simulink model "three_phase_circuit_Sim01"  (R2020b)
settings: Solver=ode4  StartTime=0.0  StopTime=inf  FixedStep=Ts  RelTol=1e-3  EnableMultiTasking=on
PostLoadFcn:
  | Ts=75e-6;
InitFcn:
  | Ts=75e-6;
undefined symbols (not defined in the file): IP, j, UDP
libraries: powerlib x40, simulink x6, powerlib_meascontrol x6, rtlab x5, rtio_generic_ip x1
Description:
  | Model of a simple control system for use iin training.
settings Model: Creator=Paul Baracos  LastModifiedBy=Antero
settings DataIOCC: LimitDataPoints=on  SaveFormat=Array  SignalLoggingSaveFormat=ModelDataLogs  SaveOutput=off  SaveTime=off  ReturnWorkspaceOutputs=off  SignalLoggingName=sigsOut
settings OptimizationCC: BlockReduction=off  BooleanDataType=off  OptimizeBlockIOStorage=off  BufferReuse=off  ExpressionFolding=off  LocalBlockOutputs=off  InitFltsAndDblsToZero=on  LifeSpan=inf
settings DebuggingCC: SaveWithParameterizedLinksMsg=none  UnderspecifiedInitializationDetection=Classic  MergeDetectMultiDrivingBlocksExec=none  SignalResolutionControl=TryResolveAllWithWarning  MultiTaskDSMMsg=warning  MultiTaskCondExecSysMsg=none  FcnCallInpInsideContextMsg=warning  SFUnexpectedBacktrackingDiag=warning  SFNoUnconditionalDefaultTransitionDiag=warning  SFExecutionAtInitializationDiag=none  ArithmeticOperatorsInVariantConditions=warning
settings HardwareCC: ProdBitPerPointer=32  ProdBitPerSizeT=32  ProdBitPerPtrDiffT=32  ProdLargestAtomicFloat=None  ProdIntDivRoundTo=Undefined  ProdEndianess=Unspecified  ProdWordSize=32  ProdHWDeviceType=32-bit Generic  TargetBitPerPointer=64  TargetBitPerSizeT=64  TargetBitPerPtrDiffT=64  TargetLongLongMode=on  TargetIntDivRoundTo=Zero  TargetEndianess=LittleEndian  TargetWordSize=64  TargetHWDeviceType=MATLAB Host  ProdEqTarget=off
settings ModelReferenceCC: PropagateSignalLabelsOutOfModel=off
settings SFSimCC: SimUseLocalCustomCode=off  CustomCodeUndefinedFunction=UseInterfaceOnly
settings RTWCC: RTWUseLocalCustomCode=off
settings CodeAppCC: StateflowObjectComments=on
settings GRTTargetCC: TargetFcnLib=ansi_tfl_tmw.mat  TargetLangStandard=C89/C90 (ANSI)  CombineOutputUpdateFcns=off  GRTInterface=on
settings ConfigComp: CovMetricSettings=dw  CovSaveCumulativeToWorkspaceVar=on  CovSaveSingleToWorkspaceVar=on  CovExternalEMLEnable=off

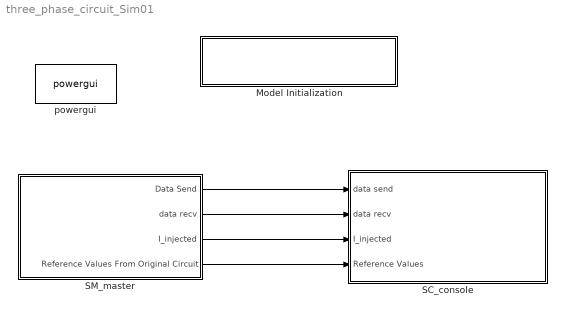
== system three_phase_circuit_Sim01 ==
  Model Initialization : Subsystem  AncestorBlock=artemis/Tools /Misc/Model Initialization  mask(Model Functions){InitFcnX=Ts=75e-6;, prel=off, posl=on, inif=on, strf=off}
      mask prompts: InitFcnX "Initialisation"; prel "Preload Function"; posl "PostLoad Function"; inif "InitFcn"; strf "StartFcn"
      mask init:
      | currentBlock = gcb;
      | root = bdroot(currentBlock);
      | 
      | if ~strcmp(get_param(root,'BlockDiagramType'),'library')
      |     if prel==1
      |         set_param(root, 'PreLoadFcn', InitFcnX);
      |     else
      |         set_param(root, 'PreLoadFcn', '');
      |     end
      |     if inif==1
      |         set_param(root, 'InitFcn', InitFcnX);
      |     else
      |         set_param(root, 'InitFcn', '');
      |     end
      |     if strf==1
      |         set_param(root, 'StartFcn', InitFcnX);
      |     else
      |         set_param(root, 'StartFcn', '');
      |     end
      |     if posl==1
      |         set_param(root, 'PostLoadFcn', InitFcnX);
      |     else
      |         set_param(root, 'PostLoadFcn', '');
      |     end
      | end
      | 
      | pos = get_param(currentBlock, 'Position');
      | width = pos(3) - pos(1); height = pos(4) - pos(2);
      | txt = [ upper(root) '\n' '- InitFcn. . . . . '  get_param(root, 'InitFcn') ];
      settings: CopyFcn=set_param(gcb,'LinkStatus','inactive')
      mask Display: text(5, height*0.5, txt, 'horizontalAlignment', 'left', 'verticalAlignment', 'middle') ;
  SC_console : Subsystem
  SM_master : Subsystem
  powergui : powerlib/powergui  Priority=1  SimulationMode=Discrete  SampleTime=Ts  frequency=60  Iterations=50  frequencyindice=60  Pbase=100e6  ErrMax=1e-4  UnitsV=kV  UnitsW=MW  buscounter=0  FunctionMessages=off  echomessages=off  EnableUseOfTLC=off  CurrentSourceSwitches=off  DisableSnubberDevices=off  DisableRonSwitches=off  DisableVfSwitches=off  DisplayEquations=off  AutomaticDiscreteSolvers=off  SolverType=Tustin/Backward Euler (TBE)  Interpol=off  ExternalGateDelay=off  methode=off  Ts=100  x0status=blocks  SPID=on  SwTol=0  HookPort=off  NonlinearTolerance=1e-4  nMaxIteration=100  ContinueOnMaxIteration=off  RestoreLinks=warning  ResistiveCurrentMeasurement=off  Frange=[0:2:500]  Ylog=off  Xlog=on  ShowGrid=off  save=off  variable=ZData  structure=0  ZoomFFT=off  StartTime=0.0  cycles=1  DisplayStyle=1  fundamental=60  FreqAxis=off  MaxFrequency=1000  frequencyindicesteady=1  RmsSteady=1  display=off
  wires:
  SM_master/1(Data Send) -> SC_console/1(data send)
  SM_master/3(I_injected) -> SC_console/3(I_injected)
  SM_master/2(data recv) -> SC_console/2(data recv)
  SM_master/4(Reference Values From Original Circuit) -> SC_console/4(Reference Values)

== system three_phase_circuit_Sim01/Model Initialization ==

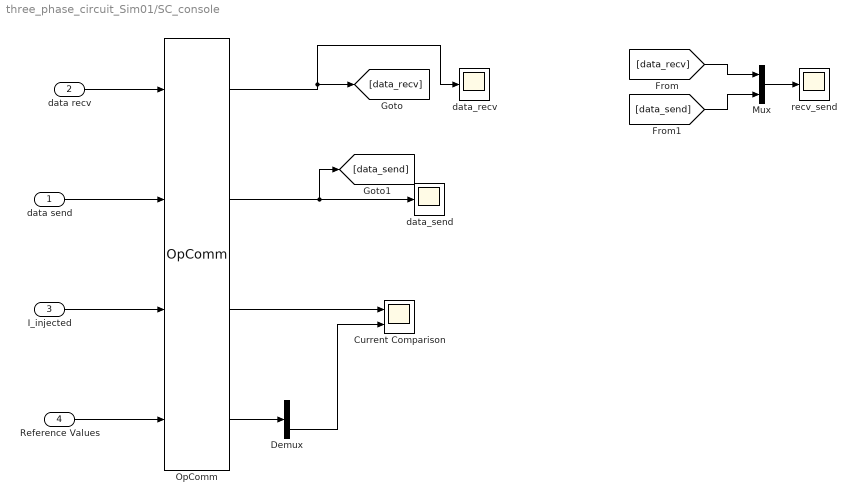
== system three_phase_circuit_Sim01/SC_console ==
  data send : Inport
  data recv : Inport  Port=2
  I_injected : Inport  Port=3
  Reference Values : Inport  Port=4
  Current Comparison : Scope  NumInputPorts=2
  Demux : Demux  Outputs=2
  Mux : Mux  Inputs=2
  OpComm : rtlab/OpComm  nbport=4  groupe_acq=1  subsys_rate=0  st=0  Synchronization=on  Interpolation=on  Threshold=1.0  Missed_Data=off  Sim_Time=off  Samples=off  dynSigOut=off  from_console=0  warning_done=off  writeOpCommFile=off  Offset=off
      settings: SourceProductName=RT-LAB
  data_recv : Scope
  data_send : Scope
  recv_send : Scope
  wires:
  OpComm/2 -> [data_send], data_send/1
  data recv/1 -> OpComm/1
  [data_recv] -> Mux/1
  OpComm/1 -> data_recv/1, [data_recv]
  Reference Values/1 -> OpComm/4
  Mux/1 -> recv_send/1
  OpComm/3 -> Current Comparison/1
  data send/1 -> OpComm/2
  I_injected/1 -> OpComm/3
  [data_send] -> Mux/2
  OpComm/4 -> Demux/1
  Demux/2 -> Current Comparison/2

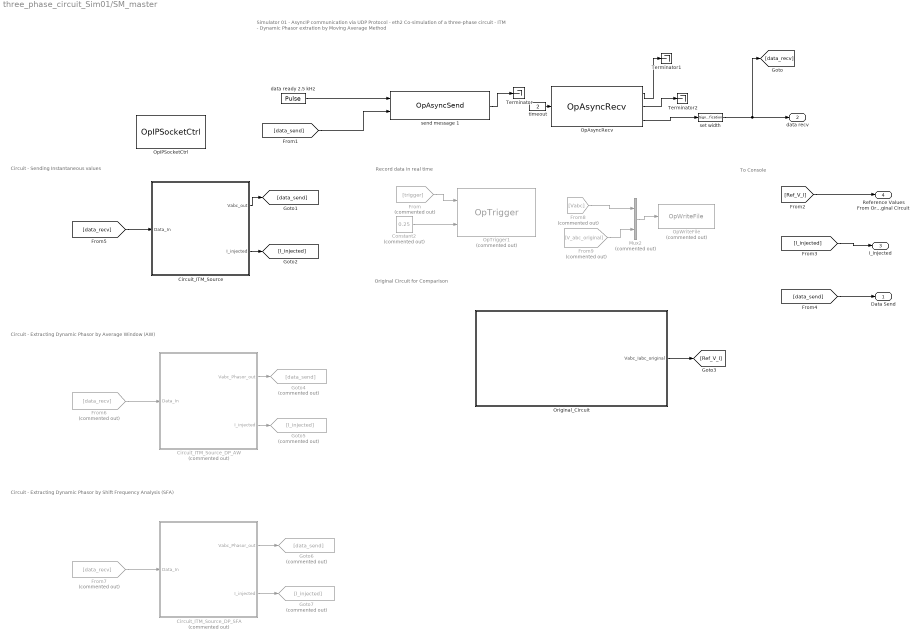
== system three_phase_circuit_Sim01/SM_master ==
  note: To Console
  note: Original Circuit for Comparison
  note: Simulator 01 - AsyncIP communication via UDP Protocol - eth2
      |
      | Co-simulation of a three-phase circuit - ITM - Dynamic Phasor extration by Moving Average Method
  note: Circuit - Sending Instantaneous values
  note: Circuit - Extracting Dynamic Phasor by Average Window (AW)
  note: Circuit - Extracting Dynamic Phasor by Shift Frequency Analysis (SFA)
  note: Record data in real time
  Circuit_ITM_Source : Subsystem
  Circuit_ITM_Source_DP_AW : Subsystem  Commented=on
  Circuit_ITM_Source_DP_SFA : Subsystem  Commented=on
  Constant2 : Constant  Commented=on  Value=0.25
  From : From  Commented=on  GotoTag=trigger
  From6 : From  Commented=on  GotoTag=data_recv
  From7 : From  Commented=on  GotoTag=data_recv
  From8 : From  Commented=on  GotoTag=Vabc
  From9 : From  Commented=on  GotoTag=V_abc_original
  Goto4 : Goto  Commented=on  GotoTag=data_send
  Goto5 : Goto  Commented=on  GotoTag=I_injected
  Goto6 : Goto  Commented=on  GotoTag=data_send
  Goto7 : Goto  Commented=on  GotoTag=I_injected
  Mux2 : Mux  Commented=on  Inputs=2
  OpAsyncRecv : rtlab/Communication/Asynchronous/OpAsyncRecv  ctl_id=1  recv_id=1  enable_param=off  fp1=1  fp2=2  fp3=3  fp4=4  fp5=5  sp1=string1  sp2=string2  sp3=string3  sp4=string4  sp5=string5  fp6=6  fp7=7
      settings: SourceProductName=RT-LAB
  OpIPSocketCtrl : rtio_generic_ip/OpIPSocketCtrl  ctl_id=1  proto=UDP/IP  ip_addr_remote=192.168.0.232  ip_port_remote=25000  ip_port_local=0  ip_addr_mcast=0.0.0.0  exe_name=AsyncIP
      settings: SourceProductName=RT-LAB I/O
  OpTrigger1 : rtlab/DataLogging/OpTrigger  Commented=on  Trig_Type=RISING EDGE  Trig_Offset=0  Acq_Group=26
      settings: SourceProductName=RT-LAB
  OpWriteFile : rtlab/DataLogging/OpWriteFile  Commented=on  Static_File=on  varname=data_voltage  Filename=data_sim02.mat  rtpath='./'  nrtpath='.\'  Acq_Group=26  file_size=8640000  write_offline=off  Sim_Mode=off  Nb_Samples=100000  Buffer_size=2400000
      settings: SourceProductName=RT-LAB
  Original_Circuit : Subsystem
  Terminator : Terminator
  Terminator1 : Terminator
  Terminator2 : Terminator
  data ready 2.5 kHz : DiscretePulseGenerator  PulseWidth=2  SampleTime=Ts
  send message 1 : rtlab/Communication/Asynchronous/OpAsyncSend  ctl_id=1  send_id=1  mode=DONT_NEED_REPLY  enable_param=off  fp1=1  fp2=2  fp3=3  fp4=4  fp5=5  sp1=string1  sp2=string2  sp3=string3  sp4=string4  sp5=string5
      settings: SourceProductName=RT-LAB
  set width : SignalSpecification  Dimensions=3  SampleTime=Ts
  timeout : Constant  Value=2
  Data Send : Outport
  data recv : Outport  Port=2
  I_injected : Outport  Port=3
  Reference Values From Original Circuit : Outport  Port=4
  wires:
  OpAsyncRecv/3 -> set width/1
  timeout/1 -> OpAsyncRecv/1
  data ready 2.5 kHz/1 -> send message 1/1
  OpAsyncRecv/1 -> Terminator1/1
  OpAsyncRecv/2 -> Terminator2/1
  set width/1 -> [data_recv], data recv/1
  [data_send] -> send message 1/2
  send message 1/1 -> Terminator/1
  [data_recv] -> Circuit_ITM_Source/1(Data_In)
  Circuit_ITM_Source/1(Vabc_out) -> [data_send]
  Circuit_ITM_Source/2(I_injected) -> [I_injected]
  [Ref_V_I] -> Reference Values From Original Circuit/1
  [I_injected] -> I_injected/1
  [data_send] -> Data Send/1
  Circuit_ITM_Source_DP_AW/2(I_injected) -> Goto5/1
  Circuit_ITM_Source_DP_AW/1(Vabc_Phasor_out) -> Goto4/1
  From6/1 -> Circuit_ITM_Source_DP_AW/1(Data_In)
  From7/1 -> Circuit_ITM_Source_DP_SFA/1(Data_In)
  Circuit_ITM_Source_DP_SFA/1(Vabc_Phasor_out) -> Goto6/1
  Original_Circuit/1(Vabc_Iabc_original) -> [Ref_V_I]
  Circuit_ITM_Source_DP_SFA/2(I_injected) -> Goto7/1
  Mux2/1 -> OpWriteFile/1
  From/1 -> OpTrigger1/1
  Constant2/1 -> OpTrigger1/2
  From9/1 -> Mux2/2
  From8/1 -> Mux2/1

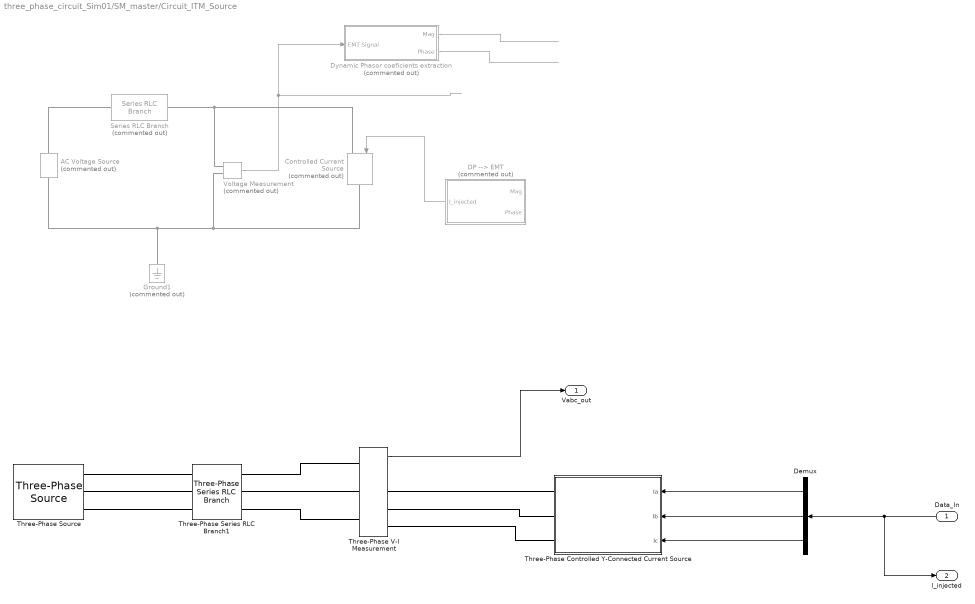
== system three_phase_circuit_Sim01/SM_master/Circuit_ITM_Source ==
  Data_In : Inport
  AC Voltage Source : powerlib/Electrical Sources/AC Voltage Source  Commented=on  Amplitude=100  Phase=0  Frequency=60  SampleTime=0  Measurements=None  BusType=swing  Pref=10e3  Qref=0  Qmin=-inf  Qmax=+inf
  Controlled Current Source : powerlib/Electrical Sources/Controlled Current Source  Commented=on  Initialize=on  Source_Type=AC  Amplitude=0  Phase=0  Frequency=0  Measurements=None
  DP --> EMT : Subsystem  Commented=on
  Demux : Demux  Outputs=3
  Dynamic Phasor coeficients extraction : Subsystem  Commented=on
  Ground1 : powerlib/Elements/Ground  Commented=on  LConnTagsString=a
  Series RLC Branch : powerlib/Elements/Series RLC Branch  Commented=on  LConnTagsString=__new0  RConnTagsString=__new0  BranchType=R  Resistance=0.5  Inductance=1e-3  SetiL0=off  InitialCurrent=0  Capacitance=1e-6  Setx0=off  InitialVoltage=0  Measurements=None
  Three-Phase Series RLC Branch1 : powerlib/Elements/Three-Phase Series RLC Branch  LConnTagsString=A|B|C  RConnTagsString=A|B|C  BranchType=R  Resistance=2  Inductance=1e-3  Capacitance=1e-6  Measurements=None
  Three-Phase V-I Measurement : powerlib/Measurements/Three-Phase V-I Measurement  VoltageMeasurement=phase-to-ground  SetLabelV=off  LabelV=Vabc  Vpu=off  VpuLL=off  CurrentMeasurement=yes  SetLabelI=off  LabelI=Iabc  Ipu=off  Pbase=100e6  Vbase=25e3  OutputType=Complex  PhasorSimulation=off  PSBequivalent=0
  Three-Phase Controlled Y-Connected Current Source : Subsystem
      settings: PortSchema="{\"entries\":[{\"content\":{\"sides\":[{\"content\":{\"connectorIds\":[\"LConn1\",\"LConn2\",\"LConn3\"]},\"type\":\"ConnectorPlacement.EquallySpacedRectSide\",\"uuid\":\"a8a67328-a09d-4495-b33c-aaf3ca0795cb\"},{\"content\":{\"connectorIds\":[\"In1\",\"In2\",\"In3\"],\"side\":\"RIGHT\"},\"type\":\"ConnectorPlacement.EquallySpacedRectSide\",\"uuid\":\"ca8d97e2-0dea-49aa-8cb7-235b4eace1f8\"},{\"content\":{\"connectorIds\":[],\"side\":\"TOP\"},\"type\":\"ConnectorPlacement.EquallySpacedRectSide\",\"uuid\":\"ab6aade9-1d27-4135-8ce1-c4358d4ecc87\"}]},\"type\":\"ConnectorPlacement.EquallySpacedConnector\",\"uuid\":\"205b5c38-55ea-4d68-a706-de660c21807c\"}],\"packageUris\":[\"http://schema.mathworks.com/mf0/Connector/19700101\"],\"version\":\"1.0\"}"
  Three-Phase Source : powerlib/Electrical Sources/Three-Phase Source  InternalConnection=Yg  VoltagePhases=off  Voltage=220  PhaseAngle=0  Voltage_phases=[25e3 25e3 25e3]/sqrt(3)  PhaseAngles_phases=[0 -120 +120]  Frequency=60  NonIdealSource=on  SpecifyImpedance=off  Resistance=0  Inductance=0  ShortCircuitLevel=100e6  BaseVoltage=220  XRratio=7  BusType=swing  Pref=10e3  Qref=0  Prefabc=[10e3, 10e3, 10e3]  Qrefabc=[0, 0, 0]  Qmin=-inf  Qmax=inf
  Voltage Measurement : powerlib/Measurements/Voltage Measurement  Commented=on  PhasorSimulation=off  OutputType=Complex  PSBequivalent=0
  Vabc_out : Outport
  I_injected : Outport  Port=2
  wires:
  DP --> EMT/1(I_injected) -> Controlled Current Source/1
  Voltage Measurement/1 -> Dynamic Phasor coeficients extraction/1(EMT Signal)
  Dynamic Phasor coeficients extraction/1(Mag) -> ?
  Dynamic Phasor coeficients extraction/2(Phase) -> ?
  Demux/1 -> Three-Phase Controlled Y-Connected Current Source/1(Ia)
  Demux/2 -> Three-Phase Controlled Y-Connected Current Source/2(Ib)
  Demux/3 -> Three-Phase Controlled Y-Connected Current Source/3(Ic)
  Data_In/1 -> Demux/1, I_injected/1
  Three-Phase V-I Measurement/1 -> Vabc_out/1
  connections:
  AC Voltage Source/RConn1 -- Series RLC Branch/LConn1
  AC Voltage Source/LConn1 -- Controlled Current Source/RConn1 -- Voltage Measurement/LConn2 -- Ground1/LConn1
  Series RLC Branch/RConn1 -- Voltage Measurement/LConn1 -- Controlled Current Source/LConn1
  Three-Phase Series RLC Branch1/LConn3 -- Three-Phase Source/RConn3
  Three-Phase Series RLC Branch1/RConn2 -- Three-Phase V-I Measurement/LConn2
  Three-Phase V-I Measurement/LConn3 -- Three-Phase Series RLC Branch1/RConn3
  Three-Phase Source/RConn1 -- Three-Phase Series RLC Branch1/LConn1
  Three-Phase V-I Measurement/LConn1 -- Three-Phase Series RLC Branch1/RConn1
  Three-Phase Source/RConn2 -- Three-Phase Series RLC Branch1/LConn2
  Three-Phase Controlled Y-Connected Current Source/LConn1 -- Three-Phase V-I Measurement/RConn1
  Three-Phase V-I Measurement/RConn2 -- Three-Phase Controlled Y-Connected Current Source/LConn2
  Three-Phase V-I Measurement/RConn3 -- Three-Phase Controlled Y-Connected Current Source/LConn3

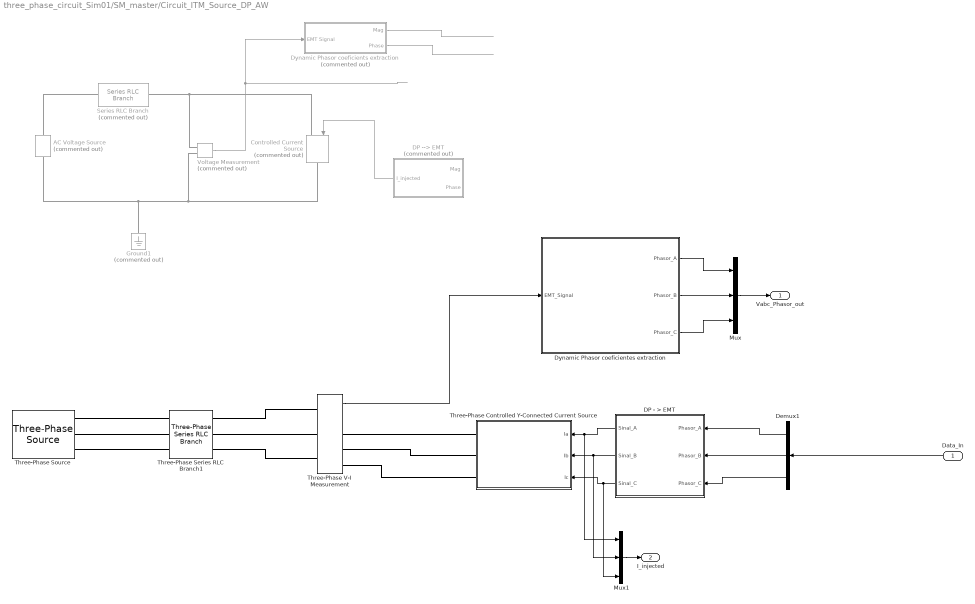
== system three_phase_circuit_Sim01/SM_master/Circuit_ITM_Source_DP_AW ==
  Data_In : Inport
  AC Voltage Source : powerlib/Electrical Sources/AC Voltage Source  Commented=on  Amplitude=100  Phase=0  Frequency=60  SampleTime=0  Measurements=None  BusType=swing  Pref=10e3  Qref=0  Qmin=-inf  Qmax=+inf
  Controlled Current Source : powerlib/Electrical Sources/Controlled Current Source  Commented=on  Initialize=on  Source_Type=AC  Amplitude=0  Phase=0  Frequency=0  Measurements=None
  DP - > EMT : Subsystem
  DP --> EMT : Subsystem  Commented=on
  Demux1 : Demux  Outputs=3
  Dynamic Phasor coeficientes extraction : Subsystem
  Dynamic Phasor coeficients extraction : Subsystem  Commented=on
  Ground1 : powerlib/Elements/Ground  Commented=on  LConnTagsString=a
  Mux : Mux  Inputs=3
  Mux1 : Mux  Inputs=3
  Series RLC Branch : powerlib/Elements/Series RLC Branch  Commented=on  LConnTagsString=__new0  RConnTagsString=__new0  BranchType=R  Resistance=0.5  Inductance=1e-3  SetiL0=off  InitialCurrent=0  Capacitance=1e-6  Setx0=off  InitialVoltage=0  Measurements=None
  Three-Phase Series RLC Branch1 : powerlib/Elements/Three-Phase Series RLC Branch  LConnTagsString=A|B|C  RConnTagsString=A|B|C  BranchType=R  Resistance=2  Inductance=1e-3  Capacitance=1e-6  Measurements=None
  Three-Phase V-I Measurement : powerlib/Measurements/Three-Phase V-I Measurement  VoltageMeasurement=phase-to-ground  SetLabelV=off  LabelV=Vabc  Vpu=off  VpuLL=off  CurrentMeasurement=yes  SetLabelI=off  LabelI=Iabc  Ipu=off  Pbase=100e6  Vbase=25e3  OutputType=Complex  PhasorSimulation=off  PSBequivalent=0
  Three-Phase Controlled Y-Connected Current Source : Subsystem
      settings: PortSchema="{\"entries\":[{\"content\":{\"sides\":[{\"content\":{\"connectorIds\":[\"LConn1\",\"LConn2\",\"LConn3\"]},\"type\":\"ConnectorPlacement.EquallySpacedRectSide\",\"uuid\":\"a8a67328-a09d-4495-b33c-aaf3ca0795cb\"},{\"content\":{\"connectorIds\":[\"In1\",\"In2\",\"In3\"],\"side\":\"RIGHT\"},\"type\":\"ConnectorPlacement.EquallySpacedRectSide\",\"uuid\":\"ca8d97e2-0dea-49aa-8cb7-235b4eace1f8\"},{\"content\":{\"connectorIds\":[],\"side\":\"TOP\"},\"type\":\"ConnectorPlacement.EquallySpacedRectSide\",\"uuid\":\"ab6aade9-1d27-4135-8ce1-c4358d4ecc87\"}]},\"type\":\"ConnectorPlacement.EquallySpacedConnector\",\"uuid\":\"205b5c38-55ea-4d68-a706-de660c21807c\"}],\"packageUris\":[\"http://schema.mathworks.com/mf0/Connector/19700101\"],\"version\":\"1.0\"}"
  Three-Phase Source : powerlib/Electrical Sources/Three-Phase Source  InternalConnection=Yg  VoltagePhases=off  Voltage=220  PhaseAngle=0  Voltage_phases=[25e3 25e3 25e3]/sqrt(3)  PhaseAngles_phases=[0 -120 +120]  Frequency=60  NonIdealSource=on  SpecifyImpedance=off  Resistance=0  Inductance=0  ShortCircuitLevel=100e6  BaseVoltage=220  XRratio=7  BusType=swing  Pref=10e3  Qref=0  Prefabc=[10e3, 10e3, 10e3]  Qrefabc=[0, 0, 0]  Qmin=-inf  Qmax=inf
  Voltage Measurement : powerlib/Measurements/Voltage Measurement  Commented=on  PhasorSimulation=off  OutputType=Complex  PSBequivalent=0
  Vabc_Phasor_out : Outport
  I_injected : Outport  Port=2
  wires:
  DP --> EMT/1(I_injected) -> Controlled Current Source/1
  Voltage Measurement/1 -> Dynamic Phasor coeficients extraction/1(EMT Signal)
  Dynamic Phasor coeficients extraction/1(Mag) -> ?
  Dynamic Phasor coeficients extraction/2(Phase) -> ?
  Data_In/1 -> Demux1/1
  Three-Phase V-I Measurement/1 -> Dynamic Phasor coeficientes extraction/1(EMT_Signal)
  Dynamic Phasor coeficientes extraction/3(Phasor_C) -> Mux/3
  Dynamic Phasor coeficientes extraction/2(Phasor_B) -> Mux/2
  Dynamic Phasor coeficientes extraction/1(Phasor_A) -> Mux/1
  Mux/1 -> Vabc_Phasor_out/1
  Demux1/1 -> DP - > EMT/1(Phasor_A)
  Demux1/2 -> DP - > EMT/2(Phasor_B)
  Demux1/3 -> DP - > EMT/3(Phasor_C)
  DP - > EMT/2(Sinal_B) -> Mux1/2, Three-Phase Controlled Y-Connected Current Source/2(Ib)
  DP - > EMT/1(Sinal_A) -> Mux1/1, Three-Phase Controlled Y-Connected Current Source/1(Ia)
  DP - > EMT/3(Sinal_C) -> Mux1/3, Three-Phase Controlled Y-Connected Current Source/3(Ic)
  Mux1/1 -> I_injected/1
  connections:
  AC Voltage Source/RConn1 -- Series RLC Branch/LConn1
  AC Voltage Source/LConn1 -- Controlled Current Source/RConn1 -- Voltage Measurement/LConn2 -- Ground1/LConn1
  Series RLC Branch/RConn1 -- Voltage Measurement/LConn1 -- Controlled Current Source/LConn1
  Three-Phase Series RLC Branch1/LConn3 -- Three-Phase Source/RConn3
  Three-Phase Series RLC Branch1/RConn2 -- Three-Phase V-I Measurement/LConn2
  Three-Phase V-I Measurement/LConn3 -- Three-Phase Series RLC Branch1/RConn3
  Three-Phase Source/RConn1 -- Three-Phase Series RLC Branch1/LConn1
  Three-Phase V-I Measurement/LConn1 -- Three-Phase Series RLC Branch1/RConn1
  Three-Phase Source/RConn2 -- Three-Phase Series RLC Branch1/LConn2
  Three-Phase Controlled Y-Connected Current Source/LConn1 -- Three-Phase V-I Measurement/RConn1
  Three-Phase V-I Measurement/RConn2 -- Three-Phase Controlled Y-Connected Current Source/LConn2
  Three-Phase V-I Measurement/RConn3 -- Three-Phase Controlled Y-Connected Current Source/LConn3

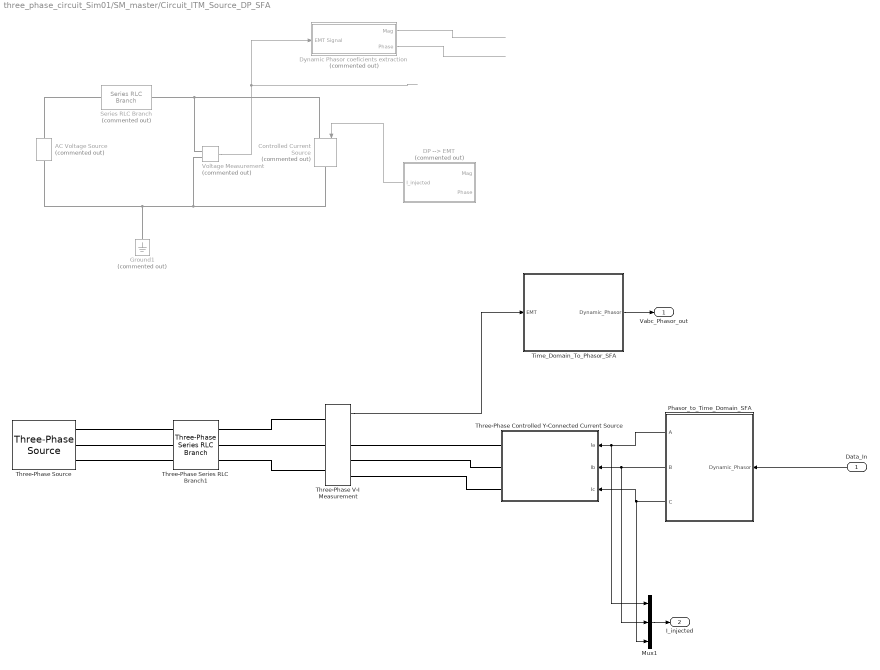
== system three_phase_circuit_Sim01/SM_master/Circuit_ITM_Source_DP_SFA ==
  Data_In : Inport
  AC Voltage Source : powerlib/Electrical Sources/AC Voltage Source  Commented=on  Amplitude=100  Phase=0  Frequency=60  SampleTime=0  Measurements=None  BusType=swing  Pref=10e3  Qref=0  Qmin=-inf  Qmax=+inf
  Controlled Current Source : powerlib/Electrical Sources/Controlled Current Source  Commented=on  Initialize=on  Source_Type=AC  Amplitude=0  Phase=0  Frequency=0  Measurements=None
  DP --> EMT : Subsystem  Commented=on
  Dynamic Phasor coeficients extraction : Subsystem  Commented=on
  Ground1 : powerlib/Elements/Ground  Commented=on  LConnTagsString=a
  Mux1 : Mux  Inputs=3
  Phasor_to_Time_Domain_SFA : Subsystem  mask(Time domain from Dynamic Phasor){offset=60}
      mask prompts: offset "Frequency shift"
      mask help: This block extracts Time Domain Signals from the Dynamic Phasor by using the SFA method. It is usable only for three-phase signals
  Series RLC Branch : powerlib/Elements/Series RLC Branch  Commented=on  LConnTagsString=__new0  RConnTagsString=__new0  BranchType=R  Resistance=0.5  Inductance=1e-3  SetiL0=off  InitialCurrent=0  Capacitance=1e-6  Setx0=off  InitialVoltage=0  Measurements=None
  Three-Phase Series RLC Branch1 : powerlib/Elements/Three-Phase Series RLC Branch  LConnTagsString=A|B|C  RConnTagsString=A|B|C  BranchType=R  Resistance=2  Inductance=1e-3  Capacitance=1e-6  Measurements=None
  Three-Phase V-I Measurement : powerlib/Measurements/Three-Phase V-I Measurement  VoltageMeasurement=phase-to-ground  SetLabelV=off  LabelV=Vabc  Vpu=off  VpuLL=off  CurrentMeasurement=yes  SetLabelI=off  LabelI=Iabc  Ipu=off  Pbase=100e6  Vbase=25e3  OutputType=Complex  PhasorSimulation=off  PSBequivalent=0
  Three-Phase Controlled Y-Connected Current Source : Subsystem
      settings: PortSchema="{\"entries\":[{\"content\":{\"sides\":[{\"content\":{\"connectorIds\":[\"LConn1\",\"LConn2\",\"LConn3\"]},\"type\":\"ConnectorPlacement.EquallySpacedRectSide\",\"uuid\":\"a8a67328-a09d-4495-b33c-aaf3ca0795cb\"},{\"content\":{\"connectorIds\":[\"In1\",\"In2\",\"In3\"],\"side\":\"RIGHT\"},\"type\":\"ConnectorPlacement.EquallySpacedRectSide\",\"uuid\":\"ca8d97e2-0dea-49aa-8cb7-235b4eace1f8\"},{\"content\":{\"connectorIds\":[],\"side\":\"TOP\"},\"type\":\"ConnectorPlacement.EquallySpacedRectSide\",\"uuid\":\"ab6aade9-1d27-4135-8ce1-c4358d4ecc87\"}]},\"type\":\"ConnectorPlacement.EquallySpacedConnector\",\"uuid\":\"205b5c38-55ea-4d68-a706-de660c21807c\"}],\"packageUris\":[\"http://schema.mathworks.com/mf0/Connector/19700101\"],\"version\":\"1.0\"}"
  Three-Phase Source : powerlib/Electrical Sources/Three-Phase Source  InternalConnection=Yg  VoltagePhases=off  Voltage=220  PhaseAngle=0  Voltage_phases=[25e3 25e3 25e3]/sqrt(3)  PhaseAngles_phases=[0 -120 +120]  Frequency=60  NonIdealSource=on  SpecifyImpedance=off  Resistance=0  Inductance=0  ShortCircuitLevel=100e6  BaseVoltage=220  XRratio=7  BusType=swing  Pref=10e3  Qref=0  Prefabc=[10e3, 10e3, 10e3]  Qrefabc=[0, 0, 0]  Qmin=-inf  Qmax=inf
  Time_Domain_To_Phasor_SFA : Subsystem  mask(SFA){offset=60}
      mask prompts: offset "Frequency shift"
      mask help: This block extracts Dynamic Phasor by using the SFA method. It is usable only for three-phase signals
  Voltage Measurement : powerlib/Measurements/Voltage Measurement  Commented=on  PhasorSimulation=off  OutputType=Complex  PSBequivalent=0
  Vabc_Phasor_out : Outport
  I_injected : Outport  Port=2
  wires:
  DP --> EMT/1(I_injected) -> Controlled Current Source/1
  Voltage Measurement/1 -> Dynamic Phasor coeficients extraction/1(EMT Signal)
  Dynamic Phasor coeficients extraction/1(Mag) -> ?
  Dynamic Phasor coeficients extraction/2(Phase) -> ?
  Data_In/1 -> Phasor_to_Time_Domain_SFA/1(Dynamic_Phasor)
  Three-Phase V-I Measurement/1 -> Time_Domain_To_Phasor_SFA/1(EMT)
  Time_Domain_To_Phasor_SFA/1(Dynamic_Phasor) -> Vabc_Phasor_out/1
  Phasor_to_Time_Domain_SFA/1(A) -> Mux1/1, Three-Phase Controlled Y-Connected Current Source/1(Ia)
  Mux1/1 -> I_injected/1
  Phasor_to_Time_Domain_SFA/2(B) -> Mux1/2, Three-Phase Controlled Y-Connected Current Source/2(Ib)
  Phasor_to_Time_Domain_SFA/3(C) -> Mux1/3, Three-Phase Controlled Y-Connected Current Source/3(Ic)
  connections:
  AC Voltage Source/RConn1 -- Series RLC Branch/LConn1
  AC Voltage Source/LConn1 -- Controlled Current Source/RConn1 -- Voltage Measurement/LConn2 -- Ground1/LConn1
  Series RLC Branch/RConn1 -- Voltage Measurement/LConn1 -- Controlled Current Source/LConn1
  Three-Phase Series RLC Branch1/LConn3 -- Three-Phase Source/RConn3
  Three-Phase Series RLC Branch1/RConn2 -- Three-Phase V-I Measurement/LConn2
  Three-Phase V-I Measurement/LConn3 -- Three-Phase Series RLC Branch1/RConn3
  Three-Phase Source/RConn1 -- Three-Phase Series RLC Branch1/LConn1
  Three-Phase V-I Measurement/LConn1 -- Three-Phase Series RLC Branch1/RConn1
  Three-Phase Source/RConn2 -- Three-Phase Series RLC Branch1/LConn2
  Three-Phase Controlled Y-Connected Current Source/LConn1 -- Three-Phase V-I Measurement/RConn1
  Three-Phase V-I Measurement/RConn2 -- Three-Phase Controlled Y-Connected Current Source/LConn2
  Three-Phase V-I Measurement/RConn3 -- Three-Phase Controlled Y-Connected Current Source/LConn3

== system three_phase_circuit_Sim01/SM_master/Original_Circuit ==
  Mux : Mux  Inputs=2
  Three-Phase Series RLC Load1 : powerlib/Elements/Three-Phase Series RLC Load  LConnTagsString=A|B|C  Configuration=Y (grounded)  NominalVoltage=25e3  Vabc=[1e3 1e3 1e3]  Vabcp=[1e3 1e3 1e3]  NominalFrequency=60  UnbalancedPower=off  ActivePower=10e6  InductivePower=200  CapacitivePower=150  Pabc=[10e3 9e3 11e3]  QLabc=[100 90 110]  QCabc=[100 90 110]  Pabcp=[10e3 9e3 11e3]  QLabcp=[100 90 110]  QCabcp=[100 90 110]  Measurements=None  LoadType=constant Z
  Three-Phase V-I Measurement1 : powerlib/Measurements/Three-Phase V-I Measurement  VoltageMeasurement=phase-to-ground  SetLabelV=off  LabelV=Vabc  Vpu=off  VpuLL=off  CurrentMeasurement=yes  SetLabelI=off  LabelI=Iabc  Ipu=off  Pbase=100e6  Vbase=25e3  OutputType=Complex  PhasorSimulation=off  PSBequivalent=0
  Three-Phase Source1 : powerlib/Electrical Sources/Three-Phase Source  InternalConnection=Yg  VoltagePhases=off  Voltage=220  PhaseAngle=0  Voltage_phases=[25e3 10e3 15e3]/sqrt(3)  PhaseAngles_phases=[40 -60 +100]  Frequency=60  NonIdealSource=on  SpecifyImpedance=off  Resistance=2  Inductance=0  ShortCircuitLevel=100e6  BaseVoltage=25e3  XRratio=7  BusType=swing  Pref=10e3  Qref=0  Prefabc=[10e3, 10e3, 10e3]  Qrefabc=[0, 0, 0]  Qmin=-inf  Qmax=inf
  Vabc_Iabc_original : Outport
  wires:
  Three-Phase V-I Measurement1/1 -> Mux/1
  Three-Phase V-I Measurement1/2 -> Mux/2
  Mux/1 -> Vabc_Iabc_original/1
  connections:
  Three-Phase V-I Measurement1/RConn2 -- Three-Phase Series RLC Load1/LConn2
  Three-Phase V-I Measurement1/RConn3 -- Three-Phase Series RLC Load1/LConn3
  Three-Phase Series RLC Load1/LConn1 -- Three-Phase V-I Measurement1/RConn1
  Three-Phase Source1/RConn2 -- Three-Phase V-I Measurement1/LConn2
  Three-Phase Source1/RConn1 -- Three-Phase V-I Measurement1/LConn1
  Three-Phase Source1/RConn3 -- Three-Phase V-I Measurement1/LConn3

== system three_phase_circuit_Sim01/SM_master/Circuit_ITM_Source/DP --> EMT ==
  Mag : Inport
  Phase : Inport  Port=2
  Compare To Constant : simulink/Logic and Bit Operations/Compare To Constant  relop=>=  const=2*pi  OutDataTypeStr=boolean
  Constant2 : Constant  Value=2*pi*60
  Integrator : Integrator  ExternalReset=rising  WrapState=on  WrappedStateUpperValue=2*pi  WrappedStateLowerValue=0  ShowStatePort=on
  Product4 : Product
  Sin3 : Trigonometry
  Sum4 : Sum  Inputs=|++
  I_injected : Outport
  wires:
  Product4/1 -> I_injected/1
  Mag/1 -> Product4/1
  Integrator/1 -> Sum4/2
  Phase/1 -> Sum4/1
  Sum4/1 -> Sin3/1
  Sin3/1 -> Product4/2
  Compare To Constant/1 -> Integrator/2
  Integrator/State -> Compare To Constant/1
  Constant2/1 -> Integrator/1

== system three_phase_circuit_Sim01/SM_master/Circuit_ITM_Source/Dynamic Phasor coeficients extraction ==
  EMT Signal : Inport
  Fourier_A : powerlib_meascontrol/Measurements/Fourier  Freq=60  n=1  InInit=[1,0]  Ts=Ts
  deg->rad : Gain  Gain=pi/180  SaturateOnIntegerOverflow=on  OutDataTypeStr=Inherit: Same as input  ParamDataTypeStr=Inherit: Same as input
  Mag : Outport
  Phase : Outport  Port=2
  wires:
  deg->rad/1 -> Phase/1
  Fourier_A/2 -> deg->rad/1
  Fourier_A/1 -> Mag/1
  EMT Signal/1 -> Fourier_A/1

== system three_phase_circuit_Sim01/SM_master/Circuit_ITM_Source/Three-Phase Controlled Y-Connected Current Source ==
  Ia : Inport
  Ib : Inport  Port=2
  Ic : Inport  Port=3
  Controlled Current Source : powerlib/Electrical Sources/Controlled Current Source  Initialize=on  Source_Type=AC  Amplitude=0  Phase=0  Frequency=0  Measurements=None
  Controlled Current Source1 : powerlib/Electrical Sources/Controlled Current Source  Initialize=on  Source_Type=AC  Amplitude=0  Phase=0  Frequency=0  Measurements=None
  Controlled Current Source2 : powerlib/Electrical Sources/Controlled Current Source  Initialize=on  Source_Type=AC  Amplitude=0  Phase=0  Frequency=0  Measurements=None
  Ground1 : powerlib/Elements/Ground  LConnTagsString=a
  A : PMIOPort  Side=Left
  B : PMIOPort  Port=2  Side=Left
  C : PMIOPort  Port=3  Side=Left
  wires:
  Ia/1 -> Controlled Current Source/1
  Ic/1 -> Controlled Current Source2/1
  Ib/1 -> Controlled Current Source1/1
  connections:
  Controlled Current Source/RConn1 -- Controlled Current Source2/RConn1 -- Ground1/LConn1 -- Controlled Current Source1/RConn1
  C/RConn1 -- Controlled Current Source2/LConn1
  B/RConn1 -- Controlled Current Source1/LConn1
  Controlled Current Source/LConn1 -- A/RConn1

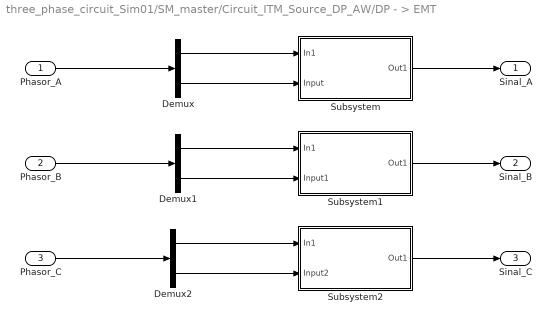
== system three_phase_circuit_Sim01/SM_master/Circuit_ITM_Source_DP_AW/DP - > EMT ==
  Phasor_A : Inport
  Phasor_B : Inport  Port=2
  Phasor_C : Inport  Port=3
  Demux : Demux  Outputs=2
  Demux1 : Demux  Outputs=2
  Demux2 : Demux  Outputs=2
  Subsystem : Subsystem
  Subsystem1 : Subsystem
  Subsystem2 : Subsystem
  Sinal_A : Outport
  Sinal_B : Outport  Port=2
  Sinal_C : Outport  Port=3
  wires:
  Subsystem2/1(Out1) -> Sinal_C/1
  Subsystem1/1(Out1) -> Sinal_B/1
  Subsystem/1(Out1) -> Sinal_A/1
  Demux/1 -> Subsystem/1(In1)
  Demux/2 -> Subsystem/2(Input)
  Demux1/1 -> Subsystem1/1(In1)
  Demux1/2 -> Subsystem1/2(Input1)
  Demux2/1 -> Subsystem2/1(In1)
  Demux2/2 -> Subsystem2/2(Input2)
  Phasor_A/1 -> Demux/1
  Phasor_B/1 -> Demux1/1
  Phasor_C/1 -> Demux2/1

== system three_phase_circuit_Sim01/SM_master/Circuit_ITM_Source_DP_AW/DP --> EMT ==
  Mag : Inport
  Phase : Inport  Port=2
  Compare To Constant : simulink/Logic and Bit Operations/Compare To Constant  relop=>=  const=2*pi  OutDataTypeStr=boolean
  Constant2 : Constant  Value=2*pi*60
  Integrator : Integrator  ExternalReset=rising  WrapState=on  WrappedStateUpperValue=2*pi  WrappedStateLowerValue=0  ShowStatePort=on
  Product4 : Product
  Sin3 : Trigonometry
  Sum4 : Sum  Inputs=|++
  I_injected : Outport
  wires:
  Product4/1 -> I_injected/1
  Mag/1 -> Product4/1
  Integrator/1 -> Sum4/2
  Phase/1 -> Sum4/1
  Sum4/1 -> Sin3/1
  Sin3/1 -> Product4/2
  Compare To Constant/1 -> Integrator/2
  Integrator/State -> Compare To Constant/1
  Constant2/1 -> Integrator/1

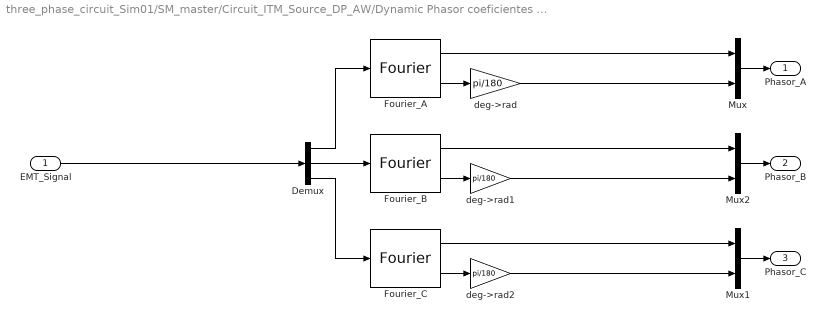
== system three_phase_circuit_Sim01/SM_master/Circuit_ITM_Source_DP_AW/Dynamic Phasor coeficientes extraction ==
  EMT_Signal : Inport
  Demux : Demux  Outputs=3
  Fourier_A : powerlib_meascontrol/Measurements/Fourier  Freq=60  n=1  InInit=[1,0]  Ts=Ts
  Fourier_B : powerlib_meascontrol/Measurements/Fourier  Freq=60  n=1  InInit=[1,-120 ]  Ts=Ts
  Fourier_C : powerlib_meascontrol/Measurements/Fourier  Freq=60  n=1  InInit=[1,+120 ]  Ts=Ts
  Mux : Mux  Inputs=2
  Mux1 : Mux  Inputs=2
  Mux2 : Mux  Inputs=2
  deg->rad : Gain  Gain=pi/180  SaturateOnIntegerOverflow=on  OutDataTypeStr=Inherit: Same as input  ParamDataTypeStr=Inherit: Same as input
  deg->rad1 : Gain  Gain=pi/180  SaturateOnIntegerOverflow=on  OutDataTypeStr=Inherit: Same as input  ParamDataTypeStr=Inherit: Same as input
  deg->rad2 : Gain  Gain=pi/180  SaturateOnIntegerOverflow=on  OutDataTypeStr=Inherit: Same as input  ParamDataTypeStr=Inherit: Same as input
  Phasor_A : Outport
  Phasor_B : Outport  Port=2
  Phasor_C : Outport  Port=3
  wires:
  Demux/2 -> Fourier_B/1
  deg->rad1/1 -> Mux2/2
  Demux/3 -> Fourier_C/1
  Demux/1 -> Fourier_A/1
  Fourier_C/1 -> Mux1/1
  EMT_Signal/1 -> Demux/1
  Fourier_B/2 -> deg->rad1/1
  deg->rad2/1 -> Mux1/2
  Fourier_A/2 -> deg->rad/1
  Fourier_C/2 -> deg->rad2/1
  Fourier_A/1 -> Mux/1
  deg->rad/1 -> Mux/2
  Fourier_B/1 -> Mux2/1
  Mux/1 -> Phasor_A/1
  Mux2/1 -> Phasor_B/1
  Mux1/1 -> Phasor_C/1

== system three_phase_circuit_Sim01/SM_master/Circuit_ITM_Source_DP_AW/Dynamic Phasor coeficients extraction ==
  EMT Signal : Inport
  Fourier_A : powerlib_meascontrol/Measurements/Fourier  Freq=60  n=1  InInit=[1,0]  Ts=Ts
  deg->rad : Gain  Gain=pi/180  SaturateOnIntegerOverflow=on  OutDataTypeStr=Inherit: Same as input  ParamDataTypeStr=Inherit: Same as input
  Mag : Outport
  Phase : Outport  Port=2
  wires:
  deg->rad/1 -> Phase/1
  Fourier_A/2 -> deg->rad/1
  Fourier_A/1 -> Mag/1
  EMT Signal/1 -> Fourier_A/1

== system three_phase_circuit_Sim01/SM_master/Circuit_ITM_Source_DP_AW/Three-Phase Controlled Y-Connected Current Source ==
  Ia : Inport
  Ib : Inport  Port=2
  Ic : Inport  Port=3
  Controlled Current Source : powerlib/Electrical Sources/Controlled Current Source  Initialize=on  Source_Type=AC  Amplitude=0  Phase=0  Frequency=0  Measurements=None
  Controlled Current Source1 : powerlib/Electrical Sources/Controlled Current Source  Initialize=on  Source_Type=AC  Amplitude=0  Phase=0  Frequency=0  Measurements=None
  Controlled Current Source2 : powerlib/Electrical Sources/Controlled Current Source  Initialize=on  Source_Type=AC  Amplitude=0  Phase=0  Frequency=0  Measurements=None
  Ground1 : powerlib/Elements/Ground  LConnTagsString=a
  A : PMIOPort  Side=Left
  B : PMIOPort  Port=2  Side=Left
  C : PMIOPort  Port=3  Side=Left
  wires:
  Ia/1 -> Controlled Current Source/1
  Ic/1 -> Controlled Current Source2/1
  Ib/1 -> Controlled Current Source1/1
  connections:
  Controlled Current Source/RConn1 -- Controlled Current Source2/RConn1 -- Ground1/LConn1 -- Controlled Current Source1/RConn1
  C/RConn1 -- Controlled Current Source2/LConn1
  B/RConn1 -- Controlled Current Source1/LConn1
  Controlled Current Source/LConn1 -- A/RConn1

== system three_phase_circuit_Sim01/SM_master/Circuit_ITM_Source_DP_SFA/DP --> EMT ==
  Mag : Inport
  Phase : Inport  Port=2
  Compare To Constant : simulink/Logic and Bit Operations/Compare To Constant  relop=>=  const=2*pi  OutDataTypeStr=boolean
  Constant2 : Constant  Value=2*pi*60
  Integrator : Integrator  ExternalReset=rising  WrapState=on  WrappedStateUpperValue=2*pi  WrappedStateLowerValue=0  ShowStatePort=on
  Product4 : Product
  Sin3 : Trigonometry
  Sum4 : Sum  Inputs=|++
  I_injected : Outport
  wires:
  Product4/1 -> I_injected/1
  Mag/1 -> Product4/1
  Integrator/1 -> Sum4/2
  Phase/1 -> Sum4/1
  Sum4/1 -> Sin3/1
  Sin3/1 -> Product4/2
  Compare To Constant/1 -> Integrator/2
  Integrator/State -> Compare To Constant/1
  Constant2/1 -> Integrator/1

== system three_phase_circuit_Sim01/SM_master/Circuit_ITM_Source_DP_SFA/Dynamic Phasor coeficients extraction ==
  EMT Signal : Inport
  Fourier_A : powerlib_meascontrol/Measurements/Fourier  Freq=60  n=1  InInit=[1,0]  Ts=Ts
  deg->rad : Gain  Gain=pi/180  SaturateOnIntegerOverflow=on  OutDataTypeStr=Inherit: Same as input  ParamDataTypeStr=Inherit: Same as input
  Mag : Outport
  Phase : Outport  Port=2
  wires:
  deg->rad/1 -> Phase/1
  Fourier_A/2 -> deg->rad/1
  Fourier_A/1 -> Mag/1
  EMT Signal/1 -> Fourier_A/1

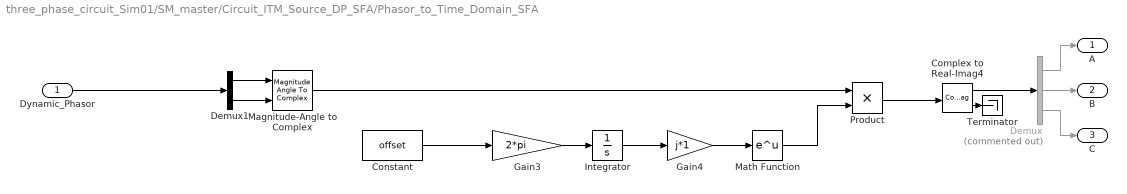
== system three_phase_circuit_Sim01/SM_master/Circuit_ITM_Source_DP_SFA/Phasor_to_Time_Domain_SFA ==
  Dynamic_Phasor : Inport
  Complex to Real-Imag4 : ComplexToRealImag
  Constant : Constant  Value=offset
  Demux : Demux  Commented=on  Outputs=3
  Demux1 : Demux  Outputs=2
  Gain3 : Gain  Gain=2*pi
  Gain4 : Gain  Gain=j*1
  Integrator : Integrator
  Magnitude-Angle to Complex : MagnitudeAngleToComplex
  Math Function : Math  SaturateOnIntegerOverflow=on
  Product : Product
  Terminator : Terminator
  A : Outport
  B : Outport  Port=2
  C : Outport  Port=3
  wires:
  Demux/2 -> B/1
  Math Function/1 -> Product/2
  Gain4/1 -> Math Function/1
  Constant/1 -> Gain3/1
  Integrator/1 -> Gain4/1
  Dynamic_Phasor/1 -> Demux1/1
  Demux/1 -> A/1
  Product/1 -> Complex to Real-Imag4/1
  Gain3/1 -> Integrator/1
  Magnitude-Angle to Complex/1 -> Product/1
  Demux/3 -> C/1
  Complex to Real-Imag4/2 -> Terminator/1
  Complex to Real-Imag4/1 -> Demux/1
  Demux1/1 -> Magnitude-Angle to Complex/1
  Demux1/2 -> Magnitude-Angle to Complex/2

== system three_phase_circuit_Sim01/SM_master/Circuit_ITM_Source_DP_SFA/Three-Phase Controlled Y-Connected Current Source ==
  Ia : Inport
  Ib : Inport  Port=2
  Ic : Inport  Port=3
  Controlled Current Source : powerlib/Electrical Sources/Controlled Current Source  Initialize=on  Source_Type=AC  Amplitude=0  Phase=0  Frequency=0  Measurements=None
  Controlled Current Source1 : powerlib/Electrical Sources/Controlled Current Source  Initialize=on  Source_Type=AC  Amplitude=0  Phase=0  Frequency=0  Measurements=None
  Controlled Current Source2 : powerlib/Electrical Sources/Controlled Current Source  Initialize=on  Source_Type=AC  Amplitude=0  Phase=0  Frequency=0  Measurements=None
  Ground1 : powerlib/Elements/Ground  LConnTagsString=a
  A : PMIOPort  Side=Left
  B : PMIOPort  Port=2  Side=Left
  C : PMIOPort  Port=3  Side=Left
  wires:
  Ia/1 -> Controlled Current Source/1
  Ic/1 -> Controlled Current Source2/1
  Ib/1 -> Controlled Current Source1/1
  connections:
  Controlled Current Source/RConn1 -- Controlled Current Source2/RConn1 -- Ground1/LConn1 -- Controlled Current Source1/RConn1
  C/RConn1 -- Controlled Current Source2/LConn1
  B/RConn1 -- Controlled Current Source1/LConn1
  Controlled Current Source/LConn1 -- A/RConn1

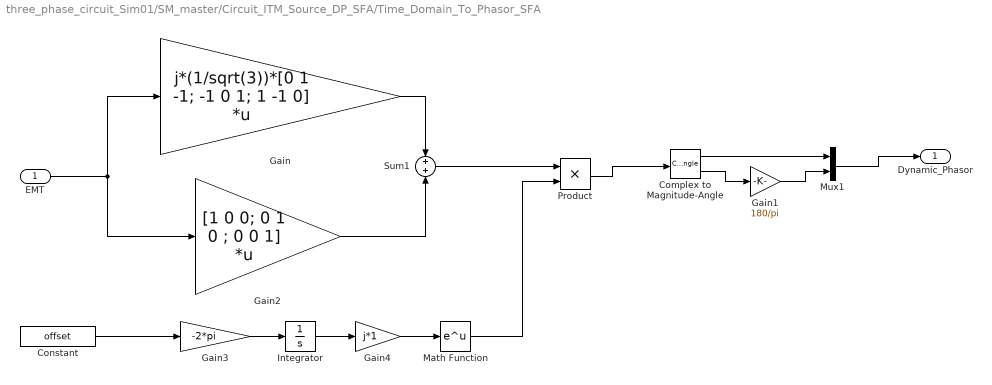
== system three_phase_circuit_Sim01/SM_master/Circuit_ITM_Source_DP_SFA/Time_Domain_To_Phasor_SFA ==
  EMT : Inport
  Complex to Magnitude-Angle : ComplexToMagnitudeAngle
  Constant : Constant  Value=offset
  Gain : Gain  Gain=j*(1/sqrt(3))*[0 1 -1; -1 0 1; 1 -1 0]  Multiplication=Matrix(K*u)
  Gain1 : Gain  Gain=180/pi
  Gain2 : Gain  Gain="[1  0 0; 0 1 0 ; 0 0 1]"  Multiplication=Matrix(K*u)
  Gain3 : Gain  Gain=-2*pi
  Gain4 : Gain  Gain=j*1
  Integrator : Integrator
  Math Function : Math  SaturateOnIntegerOverflow=on
  Mux1 : Mux  Inputs=2
  Product : Product
  Sum1 : Sum  Inputs=+|+
  Dynamic_Phasor : Outport
  wires:
  Gain3/1 -> Integrator/1
  Sum1/1 -> Product/1
  Constant/1 -> Gain3/1
  Mux1/1 -> Dynamic_Phasor/1
  Gain2/1 -> Sum1/2
  Complex to Magnitude-Angle/1 -> Mux1/1
  Gain/1 -> Sum1/1
  Gain1/1 -> Mux1/2
  EMT/1 -> Gain2/1, Gain/1
  Integrator/1 -> Gain4/1
  Math Function/1 -> Product/2
  Product/1 -> Complex to Magnitude-Angle/1
  Gain4/1 -> Math Function/1
  Complex to Magnitude-Angle/2 -> Gain1/1

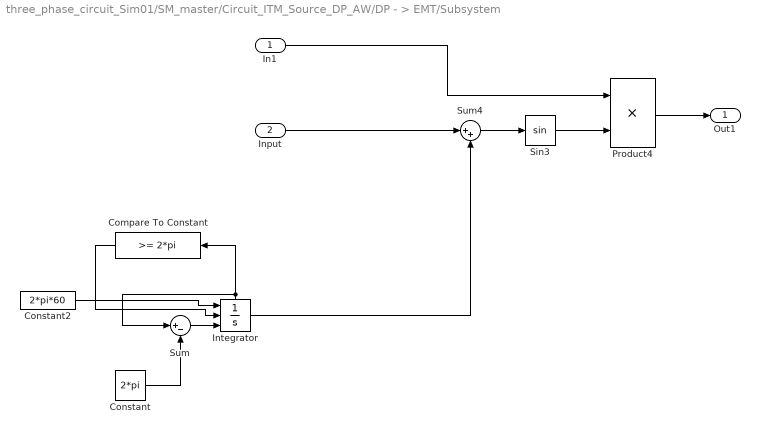
== system three_phase_circuit_Sim01/SM_master/Circuit_ITM_Source_DP_AW/DP - > EMT/Subsystem ==
  In1 : Inport
  Input : Inport  Port=2
  Compare To Constant : simulink/Logic and Bit Operations/Compare To Constant  relop=>=  const=2*pi  OutDataTypeStr=boolean
  Constant : Constant  Value=2*pi
  Constant2 : Constant  Value=2*pi*60
  Integrator : Integrator  ExternalReset=rising  InitialConditionSource=external  ShowStatePort=on
  Product4 : Product
  Sin3 : Trigonometry
  Sum : Sum  Inputs=|+-
  Sum4 : Sum  Inputs=|++
  Out1 : Outport
  wires:
  Product4/1 -> Out1/1
  In1/1 -> Product4/1
  Integrator/1 -> Sum4/2
  Input/1 -> Sum4/1
  Sum4/1 -> Sin3/1
  Sin3/1 -> Product4/2
  Integrator/State -> Sum/1, Compare To Constant/1
  Constant2/1 -> Integrator/1
  Compare To Constant/1 -> Integrator/2
  Sum/1 -> Integrator/3
  Constant/1 -> Sum/2

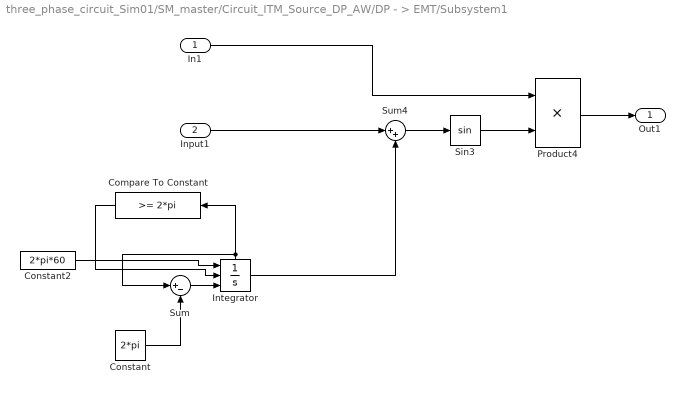
== system three_phase_circuit_Sim01/SM_master/Circuit_ITM_Source_DP_AW/DP - > EMT/Subsystem1 ==
  In1 : Inport
  Input1 : Inport  Port=2
  Compare To Constant : simulink/Logic and Bit Operations/Compare To Constant  relop=>=  const=2*pi  OutDataTypeStr=boolean
  Constant : Constant  Value=2*pi
  Constant2 : Constant  Value=2*pi*60
  Integrator : Integrator  ExternalReset=rising  InitialConditionSource=external  ShowStatePort=on
  Product4 : Product
  Sin3 : Trigonometry
  Sum : Sum  Inputs=|+-
  Sum4 : Sum  Inputs=|++
  Out1 : Outport
  wires:
  Product4/1 -> Out1/1
  In1/1 -> Product4/1
  Integrator/1 -> Sum4/2
  Input1/1 -> Sum4/1
  Sum4/1 -> Sin3/1
  Sin3/1 -> Product4/2
  Constant/1 -> Sum/2
  Sum/1 -> Integrator/3
  Compare To Constant/1 -> Integrator/2
  Integrator/State -> Sum/1, Compare To Constant/1
  Constant2/1 -> Integrator/1

== system three_phase_circuit_Sim01/SM_master/Circuit_ITM_Source_DP_AW/DP - > EMT/Subsystem2 ==
  In1 : Inport
  Input2 : Inport  Port=2
  Compare To Constant : simulink/Logic and Bit Operations/Compare To Constant  relop=>=  const=2*pi  OutDataTypeStr=boolean
  Constant : Constant  Value=2*pi
  Constant2 : Constant  Value=2*pi*60
  Integrator : Integrator  ExternalReset=rising  InitialConditionSource=external  ShowStatePort=on
  Product4 : Product
  Sin3 : Trigonometry
  Sum : Sum  Inputs=|+-
  Sum4 : Sum  Inputs=|++
  Out1 : Outport
  wires:
  Product4/1 -> Out1/1
  In1/1 -> Product4/1
  Integrator/1 -> Sum4/2
  Input2/1 -> Sum4/1
  Sum4/1 -> Sin3/1
  Sin3/1 -> Product4/2
  Integrator/State -> Sum/1, Compare To Constant/1
  Constant2/1 -> Integrator/1
  Compare To Constant/1 -> Integrator/2
  Sum/1 -> Integrator/3
  Constant/1 -> Sum/2
